simulink model "loyala"  (R2015b)
settings: Solver=VariableStepAuto  StartTime=0.0  StopTime=10  RelTol=1e-3
undefined symbols (not defined in the file): a
libraries: powerlib x35
settings Model: Creator=SPIRO  LastModifiedBy=SPIRO

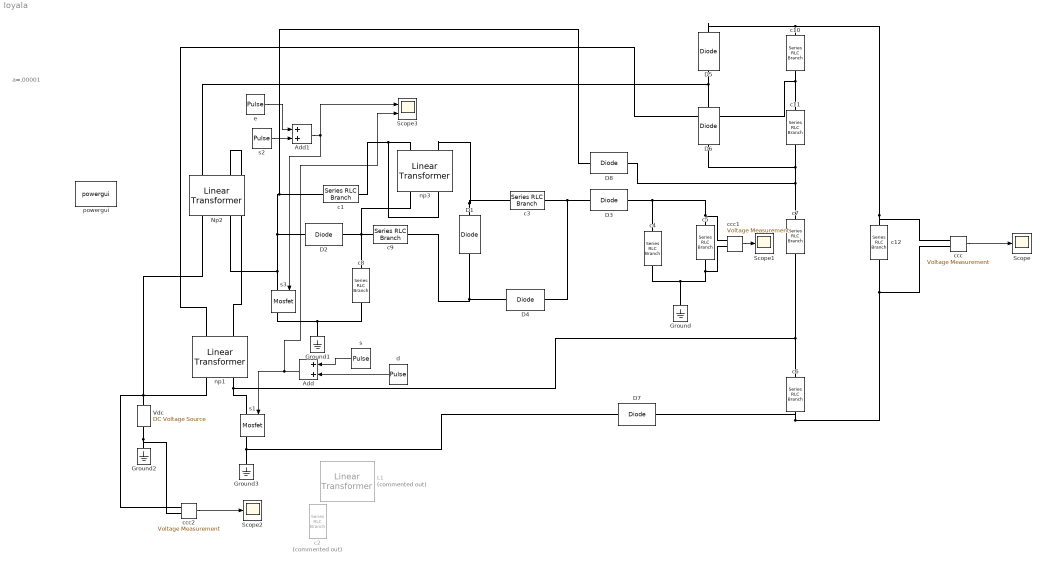
== system loyala ==
  note: a=.00001
  Add : Sum
  Add1 : Sum
  D{1..8} (8 alike) : powerlib/Power Electronics/Diode  Ron=0.001  Lon=0  Vf=0.8  IC=0  UseSnubber=off  Rs=500  Cs=250e-9  Measurements=off
  Ground{,1..3} (4 alike) : powerlib/Elements/Ground  LConnTagsString=a
  L1 : powerlib/Elements/Linear Transformer  Commented=on  UNITS=pu  NominalPower=[ 250e3 5000 ]  winding1="[ 1000  0.002  0.08 ]"  winding2="[ 1000  0.002  0.08 ]"  ThreeWindings=off  winding3=[ 315e3 0.002 0.08 ]  RmLm=[ 50 50 ]  Measurements=None  DataType=off
  Np2 : powerlib/Elements/Linear Transformer  UNITS=pu  NominalPower=[ 250e3 10000 ]  winding1="[ 1000  0.002  0.08 ]"  winding2="[ 10000 0.002  0.08 ]"  ThreeWindings=off  winding3="[ 1000  0.002  0.08 ]"  RmLm=[ 500 500 ]  Measurements=None  DataType=off
  Scope : Scope
  Scope1 : Scope
  Scope2 : Scope
  Scope3 : Scope  NumInputPorts=2
  Vdc : powerlib/Electrical Sources/DC Voltage Source  Amplitude=24  Measurements=None
  c{1,4,6..7,10..11} (6 alike) : powerlib/Elements/Series RLC Branch  LConnTagsString=__new0  RConnTagsString=__new0  BranchType=C  Resistance=1  Inductance=1e-3  SetiL0=off  InitialCurrent=0  Capacitance=1000e-6  Setx0=off  InitialVoltage=0  Measurements=None
  c12 : powerlib/Elements/Series RLC Branch  LConnTagsString=__new0  RConnTagsString=__new0  BranchType=R  Resistance=350  Inductance=1e-3  SetiL0=off  InitialCurrent=0  Capacitance=1000e-6  Setx0=off  InitialVoltage=0  Measurements=None
  c2 : powerlib/Elements/Series RLC Branch  Commented=on  LConnTagsString=__new0  RConnTagsString=__new0  BranchType=C  Resistance=1  Inductance=1e-3  SetiL0=off  InitialCurrent=0  Capacitance=1000e-6  Setx0=off  InitialVoltage=0  Measurements=None
  c3 : powerlib/Elements/Series RLC Branch  LConnTagsString=__new0  RConnTagsString=__new0  BranchType=C  Resistance=1  Inductance=1e-3  SetiL0=off  InitialCurrent=0  Capacitance=10e-6  Setx0=off  InitialVoltage=0  Measurements=None
  c5 : powerlib/Elements/Series RLC Branch  LConnTagsString=__new0  RConnTagsString=__new0  BranchType=R  Resistance=130  Inductance=1e-3  SetiL0=off  InitialCurrent=0  Capacitance=1000e-6  Setx0=off  InitialVoltage=0  Measurements=None
  c8 : powerlib/Elements/Series RLC Branch  LConnTagsString=__new0  RConnTagsString=__new0  BranchType=C  Resistance=1  Inductance=1e-3  SetiL0=off  InitialCurrent=0  Capacitance=10e-6  Setx0=off  InitialVoltage=0  Measurements=None
  c9 : powerlib/Elements/Series RLC Branch  LConnTagsString=__new0  RConnTagsString=__new0  BranchType=C  Resistance=1  Inductance=1e-3  SetiL0=off  InitialCurrent=0  Capacitance=1e-6  Setx0=off  InitialVoltage=0  Measurements=None
  ccc : powerlib/Measurements/Voltage Measurement  PhasorSimulation=off  OutputType=Complex  PSBequivalent=0
  ccc1 : powerlib/Measurements/Voltage Measurement  PhasorSimulation=off  OutputType=Complex  PSBequivalent=0
  ccc2 : powerlib/Measurements/Voltage Measurement  PhasorSimulation=off  OutputType=Complex  PSBequivalent=0
  d : DiscretePulseGenerator  PulseType=Time based  Period=.0002  PulseWidth=(70/122.5)*100  PhaseDelay=(52.5/122.5)*a
  e : DiscretePulseGenerator  PulseType=Time based  Period=a  PulseWidth=(70/122.5)*100
  np1 : powerlib/Elements/Linear Transformer  UNITS=pu  NominalPower=[ 250e3 10000 ]  winding1="[ 1000  0.002  0.08 ]"  winding2="[ 10000  0.002  0.08 ]"  ThreeWindings=off  winding3="[ 1000  0.002  0.08 ]"  RmLm=[ 500 500 ]  Measurements=None  DataType=off
  np3 : powerlib/Elements/Linear Transformer  UNITS=pu  NominalPower=[ 250e3 10000 ]  winding1="[ 1000  0.002  0.08 ]"  winding2="[ 500  0.002  0.08 ]"  ThreeWindings=off  winding3="[ 1000  0.002  0.08 ]"  RmLm=[ 500 500 ]  Measurements=None  DataType=off
  powergui : powerlib/powergui  Priority=1  SimulationMode=Discrete  SolverType=Tustin/Backward Euler (TBE)  SampleTime=5e-7  frequency=60  SPID=off  DisableSnubberDevices=off  DisableRonSwitches=off  DisableVfSwitches=off  SwTol=0  DisplayEquations=off  Interpol=off  ExternalGateDelay=off  methode=off  Ts=10  FunctionMessages=off  echomessages=off  HookPort=off  EnableUseOfTLC=off  x0status=blocks  frequencyindice=0  Pbase=100e6  ErrMax=1e-4  Iterations=50  UnitsV=kV  UnitsW=MW  buscounter=0  RestoreLinks=warning  ResistiveCurrentMeasurement=off  Frange=[0:2:500]  Ylog=off  Xlog=on  ShowGrid=off  save=off  variable=ZData  structure=0  ZoomFFT=off  StartTime=0.0  cycles=1  DisplayStyle=1  fundamental=60  FreqAxis=off  MaxFrequency=1000  frequencyindicesteady=1  RmsSteady=1  display=off
  s : DiscretePulseGenerator  PulseType=Time based  Period=a  PulseWidth=(17.5/122.5)*100
  s1 : powerlib/Power Electronics/Mosfet  Ron=0.1  Lon=0  Rd=0.01  Vfd=0  IC=0  Rs=1e5  Cs=inf  Measurements=on
  s2 : DiscretePulseGenerator  PulseType=Time based  Period=a  PulseWidth=(17.5/122.5)*100  PhaseDelay=(105/122.5)*a
  s3 : powerlib/Power Electronics/Mosfet  Ron=0.1  Lon=0  Rd=0.01  Vfd=0  IC=0  Rs=1e5  Cs=inf  Measurements=on
  wires:
  s/1 -> Add/1
  d/1 -> Add/2
  s2/1 -> Add1/2
  e/1 -> Add1/1
  Add1/1 -> s3/1, Scope3/1
  Add/1 -> Scope3/2, s1/1
  ccc/1 -> Scope/1
  ccc1/1 -> Scope1/1
  ccc2/1 -> Scope2/1
  connections:
  np1/LConn1 -- ccc2/LConn1 -- Np2/LConn1 -- Vdc/RConn1
  D2/LConn1 -- D8/LConn1 -- c1/LConn1 -- Np2/LConn2 -- s3/LConn1
  c9/RConn1 -- D1/RConn1 -- D4/LConn1
  D3/LConn1 -- D4/RConn1 -- c3/RConn1
  c4/LConn1 -- ccc1/LConn1 -- c5/LConn1 -- D3/RConn1
  c4/RConn1 -- Ground/LConn1 -- ccc1/LConn2 -- c5/RConn1
  Ground2/LConn1 -- Vdc/LConn1 -- ccc2/LConn2
  Ground3/LConn1 -- D7/RConn1 -- s1/RConn1
  c8/RConn1 -- Ground1/LConn1 -- s3/RConn1
  c8/LConn1 -- c9/LConn1 -- np3/LConn1 -- D2/RConn1
  D6/RConn1 -- Np2/RConn1 -- D5/LConn1
  c11/LConn1 -- np1/RConn1 -- c10/RConn1
  c7/LConn1 -- c11/RConn1 -- D6/LConn1 -- D8/RConn1
  s1/LConn1 -- c6/LConn1 -- c7/RConn1 -- np1/LConn2
  c6/RConn1 -- ccc/LConn2 -- c12/RConn1 -- D7/LConn1
  c12/LConn1 -- D5/RConn1 -- c10/LConn1 -- ccc/LConn1
  c1/RConn1 -- np3/LConn2 -- np3/RConn1
  c3/LConn1 -- np3/RConn2 -- D1/LConn1
  Np2/RConn2 -- np1/RConn2
